simulink model "controllers"  (R2022b)
settings: Solver=VariableStepAuto  StartTime=0.0  StopTime=0.05  RelTol=1e-3
values from neighbouring files (symbols this model uses):
  C = 125e-6    (= 0.000125)    [calculations.m]
  kp = db2mag(-6.73)    [calculations.m]
  kpd = db2mag(-42.5)    [calculations.m]
  kpi = db2mag(-4.22)    [calculations.m]
  kr = 0.2    [calculations.m]
  ku1 = round(u0/e01,1)    [calculations.m]
  L = 3.7e-4    (= 0.00037)    [calculations.m]
  rs1 = u21/i21    (= 2.33333333333)    [calculations.m]
  Td = 1/4.33e4/sqrt(0.13)    [calculations.m]
  Ti = 4/5.44e3    (= 0.000735294117647)    [calculations.m]
  u21 = round(e21-r21*i21,2)    [calculations.m]
settings Model: Creator=evely  LastModifiedBy=evely

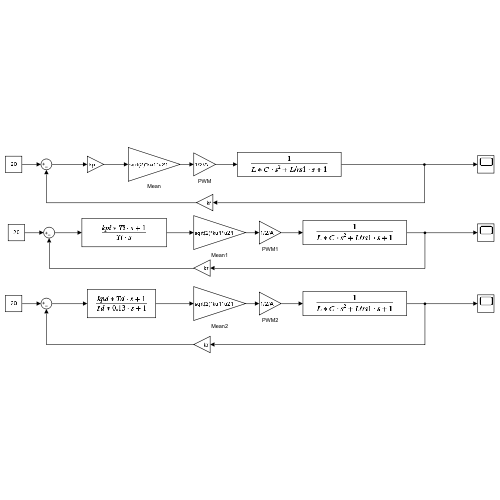
[thumbnail: Simulink's stored preview of the top-level diagram]
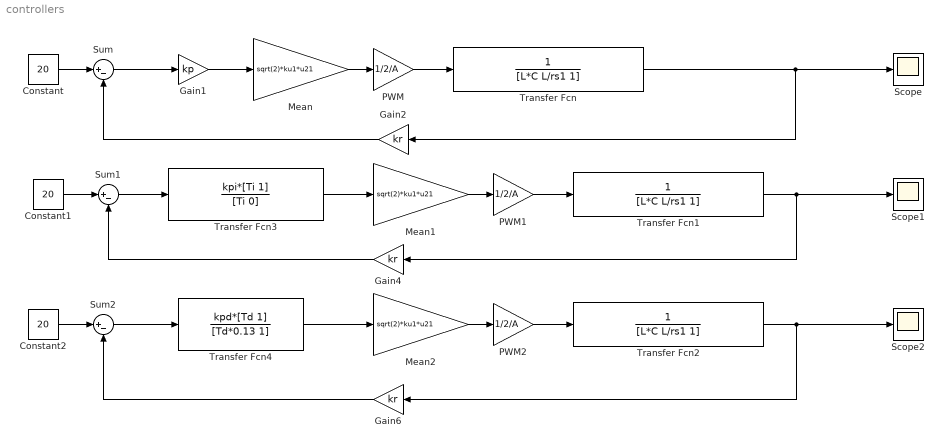
== system controllers ==
  Constant : Constant  Value=20
  Constant1 : Constant  Value=20
  Constant2 : Constant  Value=20
  Gain1 : Gain  Gain=kp
  Gain2 : Gain  Gain=kr
  Gain4 : Gain  Gain=kr
  Gain6 : Gain  Gain=kr
  Mean : Gain  Gain=sqrt(2)*ku1*u21
  Mean1 : Gain  Gain=sqrt(2)*ku1*u21
  Mean2 : Gain  Gain=sqrt(2)*ku1*u21
  PWM : Gain  Gain=1/2/A
  PWM1 : Gain  Gain=1/2/A
  PWM2 : Gain  Gain=1/2/A
  Scope : Scope
  Scope1 : Scope
  Scope2 : Scope
  Sum : Sum  Inputs=|+-
  Sum1 : Sum  Inputs=|+-
  Sum2 : Sum  Inputs=|+-
  Transfer Fcn : TransferFcn  Denominator=[L*C L/rs1 1]
  Transfer Fcn1 : TransferFcn  Denominator=[L*C L/rs1 1]
  Transfer Fcn2 : TransferFcn  Denominator=[L*C L/rs1 1]
  Transfer Fcn3 : TransferFcn  Numerator=kpi*[Ti 1]  Denominator=[Ti 0]
  Transfer Fcn4 : TransferFcn  Numerator=kpd*[Td 1]  Denominator=[Td*0.13 1]
  wires:
  Mean/1 -> PWM/1
  Constant/1 -> Sum/1
  Sum/1 -> Gain1/1
  Gain1/1 -> Mean/1
  PWM/1 -> Transfer Fcn/1
  Gain2/1 -> Sum/2
  Transfer Fcn/1 -> Gain2/1, Scope/1
  Gain4/1 -> Sum1/2
  Constant1/1 -> Sum1/1
  Transfer Fcn3/1 -> Mean1/1
  Transfer Fcn1/1 -> Gain4/1, Scope1/1
  Mean1/1 -> PWM1/1
  PWM1/1 -> Transfer Fcn1/1
  Transfer Fcn2/1 -> Gain6/1, Scope2/1
  Constant2/1 -> Sum2/1
  Transfer Fcn4/1 -> Mean2/1
  PWM2/1 -> Transfer Fcn2/1
  Gain6/1 -> Sum2/2
  Mean2/1 -> PWM2/1
  Sum1/1 -> Transfer Fcn3/1
  Sum2/1 -> Transfer Fcn4/1
